simulink model "Matpyfun"  (R2019a)
settings: Solver=VariableStepAuto  StartTime=0.0  StopTime=10.0  RelTol=1e-3
settings Model: Creator=vardhah  LastModifiedBy=vardhah

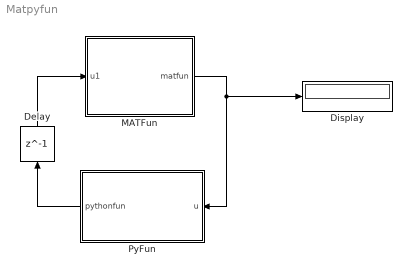
== system Matpyfun ==
  Delay : Delay  DelayLength=1  InitialCondition=0
  Display : Display
  MATFun : MATLAB Function  TreatAsAtomicUnit=on
  PyFun : MATLAB Function  TreatAsAtomicUnit=on
  wires:
  MATFun/1(matfun) -> Display/1, PyFun/1(u)
  PyFun/1(pythonfun) -> Delay/1
  Delay/1 -> MATFun/1(u1)

== matlab function Matpyfun/PyFun ==
  data: u input; pythonfun output size=1
function pythonfun = fcn(u)
pythonfun=0;
coder.extrinsic('py.testing.add_number');
pythonfun=py.testing.add_number(u);

== matlab function Matpyfun/MATFun ==
  data: u1 input; matfun output
function matfun = fcn(u1)
u2=double(u1);
matfun = u2+2;
